simulink model "SpdDemSwt_VD"  (R2016b)
settings: configuration reference "CodeGenConfigSet" (kept outside this file)
values from neighbouring files (symbols this model uses):
  SigTst_stSpdDemSwt_C = Calibration.Parameter    [init_SpdDemSwt_VD.m]
  SigTst_swtSpdDemSwt_C = Calibration.Parameter    [init_SpdDemSwt_VD.m]
undefined symbols (not defined in the file or in its folder): Switch_conv
settings Model: Creator=lenovo  LastModifiedBy=lenovo
settings ConfigSetRef: SourceLocation=Base Workspace

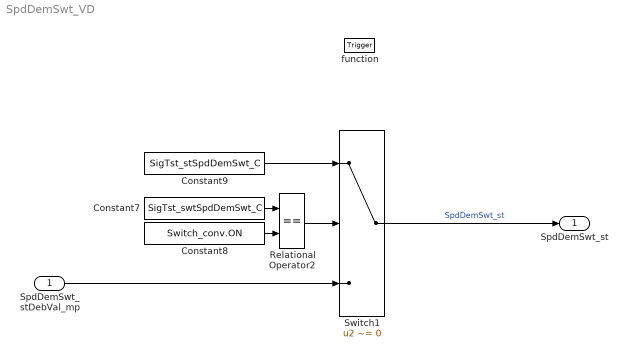
== system SpdDemSwt_VD ==
  SpdDemSwt_stDebVal_mp : Inport  Description=Debounced speed demand switch status  OutMin=0  OutMax=1  OutDataTypeStr=boolean
  function : TriggerPort  TriggerType=function-call  VariantControl=Variant
  Constant7 : Constant  Value=SigTst_swtSpdDemSwt_C
  Constant8 : Constant  Value=Switch_conv.ON
  Constant9 : Constant  Value=SigTst_stSpdDemSwt_C
  Relational Operator2 : RelationalOperator  Operator===  OutDataTypeStr=boolean  RndMeth=Nearest
  Switch1 : Switch  Criteria=u2 ~= 0  OutDataTypeStr=Inherit: Inherit via back propagation  SaturateOnIntegerOverflow=on  InputSameDT=on
  SpdDemSwt_st : Outport  Description=Speed demand switch status  OutMin=0  OutMax=1  OutDataTypeStr=boolean
  wires:
  SpdDemSwt_stDebVal_mp/1 -> Switch1/3
  Switch1/1 -> SpdDemSwt_st/1  "SpdDemSwt_st"
  Constant9/1 -> Switch1/1
  Relational Operator2/1 -> Switch1/2
  Constant7/1 -> Relational Operator2/1
  Constant8/1 -> Relational Operator2/2
